simulink model "UT2"  (R2022a)
settings: Solver=VariableStepAuto  StartTime=0.0  StopTime=72  RelTol=1e-3
settings Model: Creator=a.dehghan  LastModifiedBy=a.dehghan

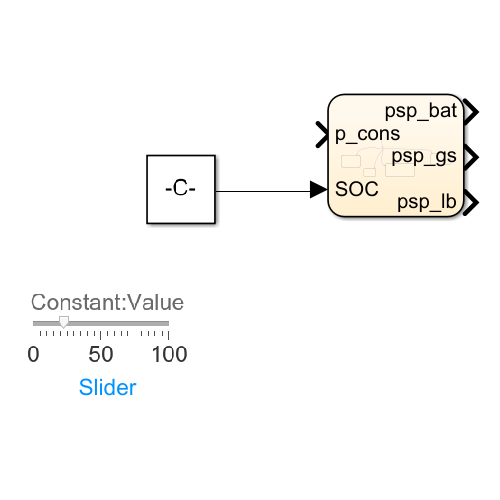
[thumbnail: Simulink's stored preview of the top-level diagram]
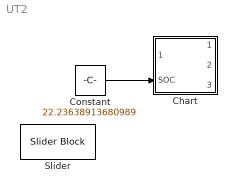
== system UT2 ==
  Chart : Stateflow chart  TreatAsAtomicUnit=on
  Constant : Constant  Value=22.23638913680989
  Slider : SliderBlock
  wires:
  Constant/1 -> Chart/2(SOC)

== stateflow chart UT2/Chart ==
  state Genset
    entry : p_cons = psp_gs;
    during :
    psp_lb = 0;
    psp_bat = 0;
  state Loadbench
    entry : p_cons = psp_lb
    during :
    psp_gs = 0;
    psp_bat = 0;
  state Battery
    entry : p_cons = psp_bat;
    during :
    psp_gs = 0;
    psp_lb = 0;
  state Exit
  (default) -> (junction 2)
  (junction 2) -> Loadbench [order 2] : [SOC > max_soc && p_cons <=0]
  (junction 2) -> Genset [order 1] : [SOC < min_soc && p_cons >=0]
  (junction 2) -> Exit [order 4]
  (junction 2) -> Battery [order 3] : [min_soc < SOC < max_soc]
  data: max_soc constant double; min_soc constant double; p_cons input; psp_bat output; psp_gs output; psp_lb output; SOC input
